simulink model "BlocksammlungJan2024_R2020"  (R2020a)
settings: Solver=ode45  StartTime=0.0  StopTime=10.0  RelTol=1e-3  EnableMultiTasking=on
undefined symbols (not defined in the file or in its folder): DiscIntNeverNeededParam, Kd, Ki, Kp, ta
libraries: simulink x13, dspxfrm3 x1
(part 1 of 2)
settings Model: Creator=METZLER  LastModifiedBy=PM
settings DataIOCC: LimitDataPoints=on  SaveFormat=Array  ReturnWorkspaceOutputs=off
settings OptimizationCC: LifeSpan=inf
settings DebuggingCC: SolverPrmCheckMsg=warning  PregeneratedLibrarySubsystemCodeDiagnostic=none  SFUnexpectedBacktrackingDiag=warning  SFNoUnconditionalDefaultTransitionDiag=warning  SFExecutionAtInitializationDiag=none  ArithmeticOperatorsInVariantConditions=warning
settings HardwareCC: ProdBitPerPointer=32  ProdBitPerSizeT=32  ProdBitPerPtrDiffT=32  ProdLargestAtomicFloat=None  ProdIntDivRoundTo=Undefined  ProdEndianess=Unspecified  ProdWordSize=32  ProdHWDeviceType=32-bit Generic
settings ModelReferenceCC: PropagateSignalLabelsOutOfModel=off
settings SFSimCC: SimUseLocalCustomCode=off  CustomCodeUndefinedFunction=UseInterfaceOnly
settings RTWCC: RTWUseLocalCustomCode=off
settings CodeAppCC: StateflowObjectComments=on
settings GRTTargetCC: TargetLangStandard=C89/C90 (ANSI)
settings ConfigComp: CovMetricSettings=dw  CovSaveCumulativeToWorkspaceVar=on  CovSaveSingleToWorkspaceVar=on  CovExternalEMLEnable=off  CovSFcnEnable=off

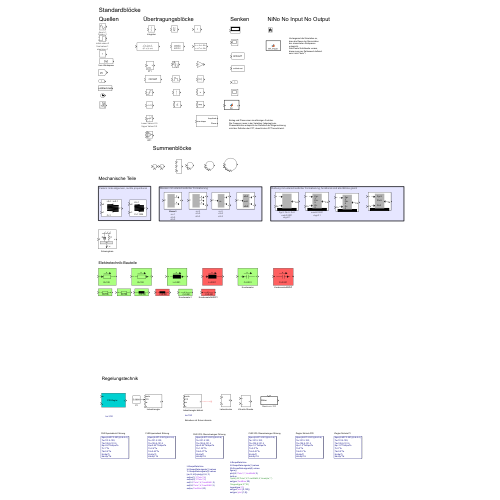
[thumbnail: Simulink's stored preview of the top-level diagram]
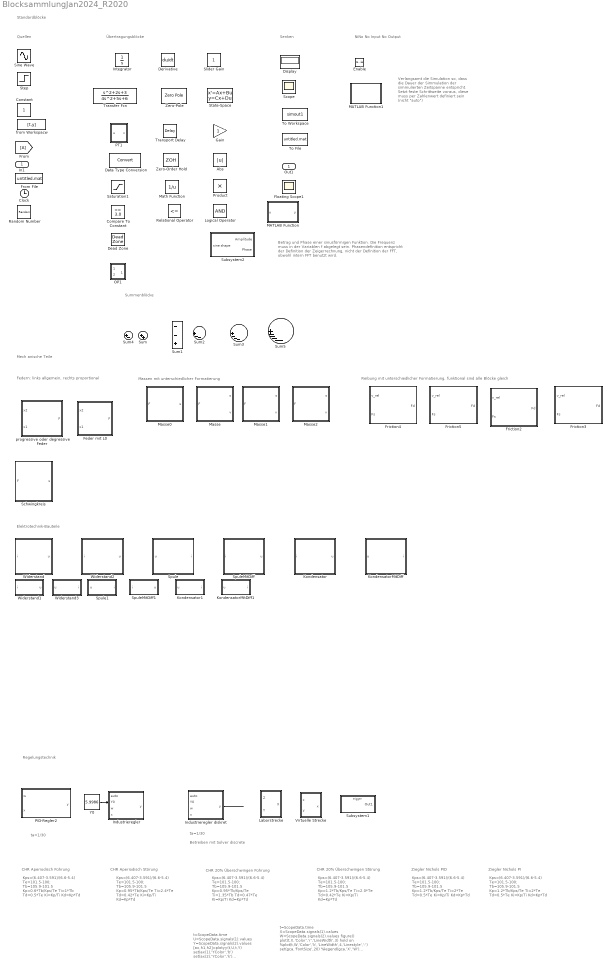
== system BlocksammlungJan2024_R2020 ==
  note: Elektrotechnik-Bauteile
  note: Federn: links allgemein, rechts proportional
  note: Reibung mit unterschiedlicher Formatierung, funktional sind alle Blöcke gleich
  note: Massen mit unterschiedlicher Formatierung
  note: Betrag und Phase einer sinusförmigen Funktion.
      | Die Frequenz muss in der Variablen f abgelegt sein.
      | Phasendefinition entspricht der Definition der Zeigerrechnung,
      | nicht der Definition der FFT, obwohl intern FFT benutzt wird.
  note: Verlangsamt die Simulation so, dass die Dauer der Simmulation der simmulierten Zeitspanne entspricht.
      | Setzt feste Schrittweite voraus, diese muss per Zahlenwert definiert sein (nicht "auto")
  note: t=ScopeData.time
      | X=ScopeData.signals(1).values
      | W=ScopeData.signals(2).values
      | figure()
      | plot(t,X,'Color','r','LineWidth',3)
      | hold on
      | %plot(t,W,'Color','k','LineWidth',4,'Linestyle',':')
      | set(gca,'FontSize',20)
      | %legend(gca,'X','W')
      | legend(gca,'X')
      | set(gca,'xlim',[0,150])
      | set(gca,'ylim',[1,8])
  note: Regelungstechnik
  note: Mech anische Teile
  note: Summenblöcke
  note: Senken
  note: Übertragungsblöcke
  note: Quellen
  note: Standardblöcke
  note: t=ScopeData.time
      | U=ScopeData.signals(1).values
      | Y=ScopeData.signals(2).values
      | [ax,h1,h2]=plotyy(t,U,t,Y)
      | set(ax(1),'YColor','b')
      | set(ax(2),'YColor','k')
      | set(h1,'Color','b','LineWidth',3)
      | set(h2,'Color','k','LineWidth',3)
      | set(ax,'FontSize',20)
  note: ta=1/30
  note: CHR Aperiodisch Führung
  note: CHR Aperiodisch Störung
  note: Kps=(6.407-3.591)/(6.6-5.4)
      | Te=101.5-100;
      | Tb=105.9-101.5
      | Kp=0.95*Tb/Kps/Te
      | Ti=1.35*Tb
      | Td=0.47*Te
      | Ki=Kp/Ti
      | Kd=Kp*Td
  note: Kps=(6.407-3.591)/(6.6-5.4)
      | Te=101.5-100;
      | Tb=105.9-101.5
      | Kp=0.6*Tb/Kps/Te
      | Ti=1*Tb
      | Td=0.5*Te
      | Ki=Kp/Ti
      | Kd=Kp*Td
  note: Kps=(6.407-3.591)/(6.6-5.4)
      | Te=101.5-100;
      | Tb=105.9-101.5
      | Kp=0.95*Tb/Kps/Te
      | Ti=2.4*Te
      | Td=0.42*Te
      | Ki=Kp/Ti
      | Kd=Kp*Td
  note: CHR 20% Überschwingen Führung
  note: Kps=(6.407-3.591)/(6.6-5.4)
      | Te=101.5-100;
      | Tb=105.9-101.5
      | Kp=1.2*Tb/Kps/Te
      | Ti=2.0*Te
      | Td=0.42*Te
      | Ki=Kp/Ti
      | Kd=Kp*Td
  note: CHR 20% Überschwingen Störung
  note: Ziegler Nichols PID
  note: Kps=(6.407-3.591)/(6.6-5.4)
      | Te=101.5-100;
      | Tb=105.9-101.5
      | Kp=1.2*Tb/Kps/Te
      | Ti=2*Te
      | Td=0.5*Te
      | Ki=Kp/Ti
      | Kd=Kp*Td
  note: NiNo No Input No Output
  note: Kps=(6.407-3.591)/(6.6-5.4)
      | Te=101.5-100;
      | Tb=105.9-101.5
      | Kp=1.2*Tb/Kps/Te
      | Ti=2*Te
      | Td=0.5*Te
      | Ki=Kp/Ti
      | Kd=Kp*Td
  note: Ziegler Nichols PI
  note: ta=1/30
  note: Betreiben mit Solver discrete
  In1 : Inport
  Enable : EnablePort
  " Feder mit L0" : Subsystem  mask{C=1.123456, L0=1}
      mask prompts: C "Spring Constant C [N/m]"; L0 "Length of Spring if no force is applied L0 [m]"
      mask help:
      | If no force F is applied, the spring has the length L0.
      |
      | F=C*sign(x2-x1-L0)*((x2-x1-L0)
      mask Display:
      | plot(20,0)
      | plot(90,100)
      | plot([60,60],[25,30])
      | plot([60,80],[30,32])
      | plot([80,40],[32,36])
      | plot([40,80],[36,40])
      | plot([80,40],[40,44])
      | plot([40,80],[44,48])
      | plot([80,40],[48,52])
      | plot([40,80],[52,56])
      | plot([80,40],[56,60])
      | plot([40,80],[60,64])
      | plot([80,40],[64,68])
      | plot([40,60],[68,70])
      | plot([60,60],[70,75])
      | 
      | 
      | port_label ('output',1,'F')
      | port_label ('input',1,'x2')
      | port_label ('input',2,'x1')
      | 
      | text(40,10,['C=',num2str(C)])
      | text(40,90,['L0=',num2str(L0)])
  " progressive oder degressive Feder" : Subsystem  mask{C=1, L0=1, Kappa=0.1}
      mask prompts: C "Federkonstante C [N/m]"; L0 "Entspannte Länge L0 [m]"; Kappa "Exponent Kappa"
      mask help:
      | Wenn keine Kraft wirkt, hat die Feder die Länge L0.
      | Progressive Feder: Kappa >0
      | Degressive Feder: Kappa <0
      | F=C*sign(x2-x1-L0)*abs(x2-x1-L0)^Kappa
      mask Display:
      | plot(20,0)
      | plot(90,100)
      | plot([60,60],[25,30])
      | plot([60,80],[30,32])
      | plot([80,40],[32,36])
      | plot([40,80],[36,40])
      | plot([80,40],[40,44])
      | plot([40,80],[44,48])
      | plot([80,40],[48,52])
      | plot([40,80],[52,56])
      | plot([80,40],[56,60])
      | plot([40,80],[60,64])
      | plot([80,40],[64,68])
      | plot([40,60],[68,70])
      | plot([60,60],[70,75])
      | 
      | 
      | port_label ('output',1,'F')
      | port_label ('input',1,'x2')
      | port_label ('input',2,'x1')
      | text(40,10,['C=',num2str(C)])
      | text(40,90,['L0=',num2str(L0),'  k=',num2str(Kappa)])
  Abs : Abs
  Clock : Clock
  Compare To Constant : simulink/Logic and Bit Operations/Compare To Constant  relop=<=  const=3.0  OutDataTypeStr=boolean
  Constant : Constant
  Data Type Conversion : DataTypeConversion
  Dead Zone : DeadZone  SaturateOnIntegerOverflow=on
      settings: AttributesFormatString=|
      | Lower Value=%<LowerValue>
      | Upper Value=%<UpperValue>
  Derivative : Derivative
  Display : Display
  Floating Scope1 : Scope
      settings: Floating=on
  Friction2 : Subsystem  mask{Fg=3, Fh=5, vhg=0.1, D=0, vsd=0.0001}
      mask prompts: Fg "Gleitreibung Fg"; Fh "Haftreibung Fh"; vhg "Übergangsbreite zwischen Haft- und Gleitreibung vhg"; D "Dämpfung D  (viskose Reibung)"; vsd "Übergangsbreite zwischen statischer und dynamischer Reibung"
      mask help:
      | Berechnet in Abhängigkeit von der Geschwindigkeit relativ zur Umgebung die Reibung eines Körpers.
      | Zunächst gibt es die statischer Reibung bei v=0 (Kraft entgegen der Summe der äußeren Kräfte ohne Fn) und die dynamische Reibung bei v<>0 (Kraft entgegen der Geschwindigkeit). Der Übergang zwischen beiden wird exponentiell verstetigt mit vsd als Übergangsbreite.
      | Dann gibt es im dynamischen noch mal einen Übergang zwischen Haftreibung (v klein) und Gleitreibung (v größer) mit vhg als Übergangsbreite. Für höhere Geschwindigkeiten macht sich noch die viskose Reibung D*v bemerkbar.
      mask Display:
      | plot(0,0)
      | plot(100,100)
      | 
      | 
      | patch([10 10 90 90],[0 10 10 0],[0 0 0 ])
      | patch([30 30 70 70],[11 90 90 11],[0.7 0.7 0.7 ])
      | plot([15 28],[75 75])
      | patch([25 25 30],[69 79 74],[0 0 0])
      | plot([71 85],[48 48])
      | patch([70 75 75],[48 43 53],[0 0 0])
      | plot([15 28],[25 25])
      | patch([25 25 30],[20 30 25],[0 0 0])
      | port_label ('output',1,'Fd')
      | port_label ('input',1,'v')
      | port_label ('input',2,'Fs')
      | text(40,80,'Fg=')
      | text(40,70,num2str(Fg))
      | %text(40,80,['Fg=',num2str(Fg)])
      | %text(40,55,['Fh=',num2str(Fh)])
      | text(40,55,'Fh=')
      | text(40,45,num2str(Fh))
      | text(40,30,'D=')
      | text(40,20,num2str(D))
  Friction3 : Subsystem  mask{Fg=3, Fh=5, vhg=0.1, D=0, vsd=0.0001}
      mask prompts: Fg "Gleitreibung Fg"; Fh "Haftreibung Fh"; vhg "Übergangsbreite zwischen Haft- und Gleitreibung vhg"; D "Dämpfung D  (viskose Reibung)"; vsd "Übergangsbreite zwischen statischer und dynamischer Reibung"
      mask help:
      | Berechnet in Abhängigkeit von der Geschwindigkeit relativ zur Umgebung die Reibung eines Körpers.
      | Zunächst gibt es die statischer Reibung bei v=0 (Kraft entgegen der Summe der äußeren Kräfte ohne Fn) und die dynamische Reibung bei v<>0 (Kraft entgegen der Geschwindigkeit). Der Übergang zwischen beiden wird exponentiell verstetigt mit vsd als Übergangsbreite.
      | Dann gibt es im dynamischen noch mal einen Übergang zwischen Haftreibung (v klein) und Gleitreibung (v größer) mit vhg als Übergangsbreite. Für höhere Geschwindigkeiten macht sich noch die viskose Reibung D*v bemerkbar.
      mask Display:
      | plot(0,0)
      | plot(100,100)
      | 
      | 
      | patch([10 10 90 90],[0 10 10 0],[0 0 0 ])
      | patch([30 30 70 70],[11 90 90 11],[0.7 0.7 0.7 ])
      | plot([15 28],[75 75])
      | patch([25 25 30],[69 79 74],[0 0 0])
      | plot([71 85],[48 48])
      | patch([70 75 75],[48 43 53],[0 0 0])
      | plot([15 28],[25 25])
      | patch([25 25 30],[20 30 25],[0 0 0])
      | port_label ('output',1,'Fd')
      | port_label ('input',1,'v')
      | port_label ('input',2,'Fs')
      | text(40,80,['Fg=',num2str(Fg)])
      | text(40,55,['Fh=',num2str(Fh)])
      | text(40,30,['D=',num2str(D)])
      | %text(40,80,'Fg=')
      | %text(40,70,num2str(Fg))
      | %text(40,55,'Fh=')
      | %text(40,45,num2str(Fh))
      | %text(40,30,'D=')
      | %text(40,20,num2str(D))
  Friction4 : Subsystem  mask{Fg=3, Fh=5, vhg=0.1, D=0, vsd=0.0001}
      mask prompts: Fg "Gleitreibung Fg"; Fh "Haftreibung Fh"; vhg "Übergangsbreite zwischen Haft- und Gleitreibung vhg"; D "Dämpfung D  (viskose Reibung)"; vsd "Übergangsbreite zwischen statischer und dynamischer Reibung"
      mask help:
      | Berechnet in Abhängigkeit von der Geschwindigkeit relativ zur Umgebung die Reibung eines Körpers.
      | Zunächst gibt es die statischer Reibung bei v=0 (Kraft entgegen der Summe der äußeren Kräfte ohne Fn) und die dynamische Reibung bei v<>0 (Kraft entgegen der Geschwindigkeit). Der Übergang zwischen beiden wird exponentiell verstetigt mit vsd als Übergangsbreite.
      | Dann gibt es im dynamischen noch mal einen Übergang zwischen Haftreibung (v klein) und Gleitreibung (v größer) mit vhg als Übergangsbreite. Für höhere Geschwindigkeiten macht sich noch die viskose Reibung D*v bemerkbar.
      settings: AttributesFormatString=|
      | Fg=%<Fg>  Fh=%<Fh>  D=%<D>\nvsd=%<vsd>
      | vhg=%<vhg>
      mask Display:
      | plot(0,0)
      | plot(100,100)
      | 
      | 
      | patch([10 10 90 90],[0 10 10 0],[0 0 0 ])
      | patch([30 30 70 70],[11 90 90 11],[0.7 0.7 0.7 ])
      | plot([15 28],[75 75])
      | patch([25 25 30],[69 79 74],[0 0 0])
      | plot([71 85],[48 48])
      | patch([70 75 75],[48 43 53],[0 0 0])
      | plot([15 28],[25 25])
      | patch([25 25 30],[20 30 25],[0 0 0])
      | port_label ('output',1,'Fd')
      | port_label ('input',1,'v')
      | port_label ('input',2,'Fs')
  Friction5 : Subsystem  mask{Fg=3, Fh=5, vhg=0.1, D=0, vsd=0.0001}
      mask prompts: Fg "Gleitreibung Fg"; Fh "Haftreibung Fh"; vhg "Übergangsbreite zwischen Haft- und Gleitreibung vhg"; D "Dämpfung D  (viskose Reibung)"; vsd "Übergangsbreite zwischen statischer und dynamischer Reibung"
      mask help:
      | Berechnet in Abhängigkeit von der Geschwindigkeit relativ zur Umgebung die Reibung eines Körpers.
      | Zunächst gibt es die statischer Reibung bei v=0 (Kraft entgegen der Summe der äußeren Kräfte ohne Fn) und die dynamische Reibung bei v<>0 (Kraft entgegen der Geschwindigkeit). Der Übergang zwischen beiden wird exponentiell verstetigt mit vsd als Übergangsbreite.
      | Dann gibt es im dynamischen noch mal einen Übergang zwischen Haftreibung (v klein) und Gleitreibung (v größer) mit vhg als Übergangsbreite. Für höhere Geschwindigkeiten macht sich noch die viskose Reibung D*v bemerkbar.
      settings: AttributesFormatString=|
      | nvsd=%<vsd>
      | vhg=%<vhg>
      mask Display:
      | plot(0,0)
      | plot(100,100)
      | 
      | 
      | patch([10 10 90 90],[0 10 10 0],[0 0 0 ])
      | patch([30 30 70 70],[11 90 90 11],[0.7 0.7 0.7 ])
      | plot([15 28],[75 75])
      | patch([25 25 30],[69 79 74],[0 0 0])
      | plot([71 85],[48 48])
      | patch([70 75 75],[48 43 53],[0 0 0])
      | plot([15 28],[25 25])
      | patch([25 25 30],[20 30 25],[0 0 0])
      | port_label ('output',1,'Fd')
      | port_label ('input',1,'v')
      | port_label ('input',2,'Fs')
      | text(40,80,'Fg=')
      | text(40,70,num2str(Fg))
      | %text(40,80,['Fg=',num2str(Fg)])
      | %text(40,55,['Fh=',num2str(Fh)])
      | text(40,55,'Fh=')
      | text(40,45,num2str(Fh))
      | text(40,30,'D=')
      | text(40,20,num2str(D))
  From File : FromFile  SampleTime=0
  Gain : Gain
  Industrieregler : Subsystem  mask{Kp=Kp, Ki=Ki, Kd=Kd, T=0.1, Ts=0.1, E0_auf_I=on, E0_auf_P=on, Stossfrei=on}
      mask prompts: T "Zeitkonstante   DT1-Glied"; Ts "Dauer Ts der stossfreien Umschaltung (>0)"; E0_auf_I "Integrier-Pfad sieht Anfangsfehler"; E0_auf_P "Proportional-Pfad sieht Anfangsfehler"; Stossfrei "Stossfreie Umschaltung"
      mask help:
      | Industrieregler. Zum Korrekten Hin- und Herschalten zwischen Hand und Automatik muss Y0 aus einer Konstantquelle namens Y0 kommen,
      | Diese Variante funktioniert auch mit variabler Schrittweite.
      | Wegen den kontinuierlichen Zuständen funktioniert diese Variante aber nicht mit Hardwaretargets.
      mask Display:
      | port_label('input',1,'auto');
      | port_label('input',2,'Y0');
      | port_label('input',3,'w');
      | port_label('input',4,'x');
      | port_label('output',1,'y');
  Industrieregler diskret : Subsystem  mask{Kp=0.885, Ki=0.17, Kd=0.99, T=1, Ts=1, E0_auf_I=on, E0_auf_P=off, Stossfrei=on}
      mask prompts: T "Zeitkonstante   DT1-Glied"; Ts "Dauer Ts der stossfreien Umschaltung (>0)"; E0_auf_I "Integrier-Pfad sieht Anfangsfehler"; E0_auf_P "Proportional-Pfad sieht Anfangsfehler"; Stossfrei "Stossfreie Umschaltung"
      mask help:
      | Industrieregler.
      | Zum Korrekten Hin- und Herschalten zwischen Hand und Automatik muss Y0 aus einer Konstantquelle namens Y0 kommen,
      | Diese Variante funktioniertnur mit fester Schrittweite.
      | Diese Variante funktioniert auch mit Hardwaretargets.
      mask Display:
      | port_label('input',1,'auto');
      | port_label('input',2,'Y0');
      | port_label('input',3,'w');
      | port_label('input',4,'x');
      | port_label('output',1,'y');
  Integrator : Integrator
  Kondensator : Subsystem  mask{C=1E-3}
      mask prompts: C "Kappazität C [F]"
      mask help:
      | Kapazität
      | Eingang ist u, Ausgang ist i.
      | i=1/C * integral(u)
      mask Display:
      | plot(0,0)
      | plot(100,100)
      | plot([0 0],[1 1]) %Umschalten auf dicke Linien
      | %patch([30 30 70 70 30],[40 60 60 40 40],[0,0,0])
      | plot([45 45],[40 60])
      | plot([55 55],[40 60])
      | plot([15 45],[50 50])
      | patch([25,32,25],[45,50,55],[0,0,0])
      | plot([55 85],[50 50])
      | plot([30 70],[70 70])
      | patch([63 70 63],[65 70 75], [0,0,0])
      | text(45,80,['u'])
      | 
      | text(30,20,['C=',num2str(C)])
      | 
      | 
      | 
      | port_label ('output',1,'u')
      | port_label ('input',1,'i')
  Kondensator1 : Subsystem  mask{C=1E-3}
      mask prompts: C "Kappazität C [F]"
      mask help:
      | Kapazität
      | Eingang ist u, Ausgang ist i.
      | i=1/C * integral(u)
      mask Display:
      | plot(0,0)
      | plot(100,100)
      | plot([0 0],[1 1]) %Umschalten auf dicke Linien
      | %patch([30 30 70 70 30],[40 60 60 40 40],[0,0,0])
      | plot([45 45],[40 60])
      | plot([55 55],[40 60])
      | plot([15 45],[50 50])
      | 
      | plot([55 85],[50 50])
      | 
      | 
      | 
      | text(30,19,['C=',num2str(C)])
      | 
      | 
      | 
      | port_label ('output',1,'u')
      | port_label ('input',1,'i')
  KondensatorMitDiff : Subsystem  mask{C=1E-3}
      mask prompts: C "Kappazität C [F]"
      mask help:
      | Kapazität
      | Eingang ist u, Ausgang ist i.
      | i=C*u'
      | Wegen Diff-Block nicht für jeden Solver geeignet.
      mask Display:
      | plot(0,0)
      | plot(100,100)
      | plot([0 0],[1 1]) %Umschalten auf dicke Linien
      | %patch([30 30 70 70 30],[40 60 60 40 40],[0,0,0])
      | plot([45 45],[40 60])
      | plot([55 55],[40 60])
      | plot([15 45],[50 50])
      | patch([70,77,70],[45,50,55],[0,0,0])
      | plot([55 85],[50 50])
      | plot([30 70],[70 70])
      | patch([63 70 63],[65 70 75], [0,0,0])
      | text(45,80,['u'])
      | 
      | text(30,20,['C=',num2str(C)])
      | 
      | 
      | 
      | port_label ('output',1,'i')
      | port_label ('input',1,'u')
  KondensatorMitDiff1 : Subsystem  mask{C=1E-3}
      mask prompts: C "Kappazität C [F]"
      mask help:
      | Kapazität
      | Eingang ist u, Ausgang ist i.
      | i=C*u'
      | Wegen Diff-Block nicht für jeden Solver geeignet.
      mask Display:
      | plot(0,0)
      | plot(100,100)
      | plot([0 0],[1 1]) %Umschalten auf dicke Linien
      | %patch([30 30 70 70 30],[40 60 60 40 40],[0,0,0])
      | plot([45 45],[40 60])
      | plot([55 55],[40 60])
      | plot([15 45],[50 50])
      | 
      | plot([55 85],[50 50])
      | 
      | 
      | 
      | text(30,19,['C=',num2str(C)])
      | 
      | 
      | 
      | port_label ('output',1,'i')
      | port_label ('input',1,'u')
  Laborstrecke : Subsystem
  Logical Operator : Logic  AllPortsSameDT=off  OutDataTypeStr=boolean
  MATLAB Function : MATLAB Function  TreatAsAtomicUnit=on
  MATLAB Function1 : MATLAB Function  TreatAsAtomicUnit=on
  Masse : Subsystem  mask{m=2, v0=0, s0=3}
      mask prompts: m "Masse m"; v0 "Anfangsgeschwindigkeit v_0"; s0 "Anfangsposition s_0"
      mask help:
      | Calculates the position s and the velocity v of a mass as a function of the Force F and the initial velocity v_0 and initial position s_0.
      | Berechnet die Position und die Geschwindigkeit eines Köpers mit der Masse m. Auf den Köper wirkt die Kraft F. Die Anfangsposition ist s_0, die Anfangsgeschwindigkeit ist v_0.
      settings: AttributesFormatString=m=%<m>\nv0=%<v0>\ns0=%<s0>
      mask Display:
      | plot(0,0)
      | plot(100,100)
      | patch([20 20 60 60],[10 90 90 10],[0.7,0.7,0.7])
      | plot([60 80],[70 70])
      | patch([80 80 85],[65 75 70],[0 0 0])
      | text(70,80,'s')
      | plot([60 80],[50 50])
      | patch([80 80 85],[45 55 50],[0 0 0])
      | text(70,60,'F')
      | plot([60 80],[30 30])
      | patch([80 80 85],[25 35 30],[0 0 0])
      | text(70,40,'v')
      | port_label ('output',1,'s')
      | port_label ('output',2,'v')
      | port_label ('input',1,'F')
  Masse0 : Subsystem  mask(Starrer Körper){m=1, v0=0, s0=0}
      mask prompts: m "Masse m"; v0 "Anfangsgeschwindigkeit v0"; s0 "Anfangsposition s0"
      mask help: Berechnet die Position eines Körpers als Funktion der auf ihn wirkenden Kraft F, seiner Masse m, der Anfangsgeschwindigkeit v0 und der Anfangsposition s0.
      settings: AttributesFormatString=m=%<m>\nv0=%<v0>\ns0=%<s0>
      mask Help:
      | Die Position x eines starren Körpers der Masse m berechnet sich aus:
      | F=m*X''
      | 
      | Erstellt von Patrick Metzler für Hochschule RheinMain.
      mask Display:
      | plot(0,0)
      | plot(100,100)
      | patch([20 20 60 60],[10 90 90 10],[0.7,0.7,0.7])
      | plot([60 80],[70 70])
      | patch([80 80 85],[65 75 70],[0 0 0])
      | text(70,80,'F')
      | plot([60 80],[30 30])
      | patch([80 80 85],[25 35 30],[0 0 0])
      | text(70,40,'s')
      | port_label ('output',1,'s')
      | port_label ('input',1,'F')
  Masse1 : Subsystem  mask{m=2, v0=0, s0=3}
      mask prompts: m "Masse m"; v0 "Anfangsgeschwindigkeit v_0"; s0 "Anfangsposition s_0"
      mask help:
      | Calculates the position s and the velocity v of a mass as a function of the Force F and the initial velocity v_0 and initial position s_0.
      | Berechnet die Position und die Geschwindigkeit eines Köpers mit der Masse m. Auf den Köper wirkt die Kraft F. Die Anfangsposition ist s_0, die Anfangsgeschwindigkeit ist v_0.
      settings: AttributesFormatString=m=%<m>\nv0=%<v0>\ns0=%<s0>
      mask Display:
      | plot(0,0)
      | plot(100,100)
      | patch([35 35 70 70],[10 90 90 10],[0.7,0.7,0.7])
      | text(45,50,'m')
      | plot([70 80],[70 70])
      | patch([80 80 85],[65 75 70],[0 0 0])
      | plot([15 35],[50 50])
      | patch([30 30 35],[45 55 50],[0 0 0])
      | plot([70 80],[30 30])
      | patch([80 80 85],[25 35 30],[0 0 0])
      | port_label ('output',1,'s')
      | port_label ('output',2,'v')
      | port_label ('input',1,'F')
  Masse2 : Subsystem  mask{m=2, v0=0, s0=3}
      mask prompts: m "Masse m"; v0 "Anfangsgeschwindigkeit v_0"; s0 "Anfangsposition s_0"
      mask help:
      | Calculates the position s and the velocity v of a mass as a function of the Force F and the initial velocity v_0 and initial position s_0.
      | Berechnet die Position und die Geschwindigkeit eines Köpers mit der Masse m. Auf den Köper wirkt die Kraft F. Die Anfangsposition ist s_0, die Anfangsgeschwindigkeit ist v_0.
      mask Display:
      | plot(0,0)
      | plot(100,100)
      | patch([35 35 70 70],[10 90 90 10],[0.7,0.7,0.7])
      | text(40,80,['s0=',num2str(s0)])
      | text(40,50,['m=',num2str(m)])
      | text(40,20,['v0=',num2str(v0)])
      | plot([70 80],[70 70])
      | patch([80 80 85],[65 75 70],[0 0 0])
      | plot([15 35],[50 50])
      | patch([30 30 35],[45 55 50],[0 0 0])
      | plot([70 80],[30 30])
      | patch([80 80 85],[25 35 30],[0 0 0])
      | port_label ('output',1,'s')
      | port_label ('output',2,'v')
      | port_label ('input',1,'F')
  Math Function : Math  Operator=reciprocal  SignedPower=on  SaturateOnIntegerOverflow=on
  OP1 : Subsystem  mask{k0=1E5, fg=100000}
      mask prompts: k0 "Open Loop Gain [V/V]"; fg "Open Loop Band Width [Hz]"
      mask init:
      | set_param(gcb,'MaskHideContents','off')
      mask Display:
      | color('black')
      | patch([0.2 0.2 0.8 0.2],[0.05 0.95 0.5 0.051],[0.9 0.9 0.9 ])
      | plot([0.2 0.2],[0.05 0.95])% Senkrecht Gehäuse
      | 
      | plot([0.2 0.8],[0.95 0.5])% Gehäuse oben schräg
      | plot([0.2 0.8],[0.051 0.5])% Gehäuse unten schräg
      | plot([0.0 0.2],[0.75 0.75])% Leiterbahn Plus
      | plot([0.0 0.2],[0.25 0.25])% Leiterbahn Minus
      | plot([0.8 1],[0.5 0.5])% Leiterbahn ua
      | text(0.29,0.76,'+')
      | text(0.29,0.28,'-')
      | %patch([0.1 0.9 0.9 0.1 0.1],[0.1 0.1 0.9 0.9 0.1],[0 0 0 ])
  PID-Regler2 : Subsystem  mask{Kp=1, Ki=1, Kd=1, T=0.1}
      mask prompts: T "T  Zeitkonstante des PT1-Glieds vor dem D-Glied"
      mask help: Ein einfacher PID-Regler
      mask Display:
      | IconText='';
      | if ~strcmp(get_param(gcb,'Kp'),'0')
      |     IconText=strcat(IconText,'P');
      | end
      | if ~strcmp(get_param(gcb,'Ki'),'0')
      |    IconText=strcat(IconText,'I');
      | end
      | if ~strcmp(get_param(gcb,'Kd'),'0')
      |     IconText=strcat(IconText,'D');
      | end
      | IconText=strcat(IconText,'-Regler')
      | plot(0,0)
      | plot(100,100)
      | text(25,50,IconText)
      | port_label ('output',1,'y')
      | port_label ('input',1,'w')
      | port_label ('input',2,'x')
  PT1 : Subsystem  mask{k=1, T=1}
      mask prompts: k "Verstärkung"; T "Zeitkonstante"
      mask help: PT1-Glied
      mask Display:
      | plot(0,0)
      | plot(100,100)
      | text(20,20,'PT1')
      | port_label ('output',1,'v')
      | port_label ('input',1,'u')
  Product : Product
  Random Number : RandomNumber  SampleTime=0.1
  Relational Operator : RelationalOperator  Operator=<=  OutDataTypeStr=boolean  RndMeth=Simplest
  Saturation1 : Saturate
  Schwingkreis : Subsystem  mask{v0=0, C=1, D=1, m=1}
      mask prompts: v0 "Anfangsgeschwindigkeit [m/s]"; C "Federkonstante [N/m]"; D "Dämpfung [Ns/m]"; m "Masse [kg]"
      mask help:
      | Ein einfacher Schwingkreis erregt durch die Kraft F antwortet mit der Position x.
      | Die Kraft wird in Newton erwartet, die Position wird in Metern ausgegeben.
      mask Display:
      | plot(0,0)
      | plot(100,100)
      | %innerhalb einer Make hat das plot-commando
      | %keine modifier.
      | %Durch zweimal gleiche Koordinaten am Anfang des
      | %plot-Kommandos wird auf dicke Linie umgeschaltet.
      | 
      | plot([20,20 70],[80,80 80])
      | plot([30 40],[80 90])
      | plot([45 55],[80 90])
      | plot([60 70],[80 90])
      | 
      | patch([30 42 42 30],[55 55 58 58],[0 0 0 ])
      | plot([28 28],[63 50])
      | plot([42 42],[63 50])
      | plot([28 42],[50 50])
      | plot([35 35],[60 80])
      | plot([35 35],[50 30])
      | 
      | patch([14 78 78 14],[26 26 38 38],[0.9 0.9 0.9])
      | text(44,33,'m')
      | plot([10 80],[25 25])
      | plot([10 80],[39 39])
      | plot([10 10],[25 39])
      | plot([80 80],[25 39])
      | 
      | plot([60 60],[80 70])
      | plot([60 55],[70 68])
      | plot([55 65],[68 64])
      | plot([65 55],[64 60])
      | plot([55 65],[60 55])
      | plot([55 65],[51 55])
      | plot([55 60],[51 49])
      | plot([60 60],[49 39])
      | 
      | plot([45 45],[25 5])
      | 
      | patch([43 46 49],[10 5 10],[0  0 0])
      | 
      | text(50,15,'F, x')
      | text(70,60,'C')
      | text(20,60,'D')
      | 
      | port_label ('output',1,'x')
      | port_label ('input',1,'F')
  Scope : Scope
  Sine Wave : Sin  SampleTime=0
      settings: AttributesFormatString=|
      | Ampl.=%<Amplitude>
      | Frequ.=%<Frequency>
      | Offset=%<Offset>
      | Phase=%<Phase>
  Slider Gain : simulink/Math Operations/Slider Gain  gain=1  low=0  high=2
  Spule : Subsystem  mask{L=1E-3}
      mask prompts: L "Induktivität L [H]"
      mask help:
      | Induktivität:
      | Eingang ist u, Ausgang ist i.
      mask Display:
      | plot(0,0)
      | plot(100,100)
      | plot([0 0],[1 1]) %Umschalten auf dicke Linien
      | patch([30 30 70 70 30],[40 60 60 40 40],[0,0,0])
      | plot([15 30],[50 50])
      | patch([75,82,75],[45,50,55],[0,0,0])
      | plot([70 88],[50 50])
      | plot([30 70],[70 70])
      | patch([63 70 63],[65 70 75], [0,0,0])
      | text(45,80,['u'])
      | 
      | text(30,20,['L=',num2str(L)])
      | 
      | 
      | 
      | port_label ('output',1,'i')
      | port_label ('input',1,'u')
  Spule1 : Subsystem  mask{L=1E-3}
      mask prompts: L "Induktivität L [H]"
      mask help:
      | Induktivität:
      | Eingang ist u, Ausgang ist i.
      mask Display:
      | plot(0,0)
      | plot(100,100)
      | plot([0 0],[1 1]) %Umschalten auf dicke Linien
      | patch([30 30 70 70 30],[35 65 65 35 35],[0,0,0])
      | plot([15 30],[50 50])
      | plot([70 88],[50 50])
      | text(30,20,['L=',num2str(L)])
      | port_label ('output',1,'i')
      | port_label ('input',1,'u')
  SpuleMitDiff : Subsystem  mask{L=1E-3}
      mask prompts: L "Induktivität L [H]"
      mask help:
      | Induktivität
      | Eingang ist i, Ausgang ist u.
      | u=L*i'
      | Wegen Diff-Block nicht für alle Solver geeignet.
      mask Display:
      | plot(0,0)
      | plot(100,100)
      | plot([0 0],[1 1]) %Umschalten auf dicke Linien
      | patch([30 30 70 70 30],[40 60 60 40 40],[0,0,0])
      | plot([15 30],[50 50])
      | patch([20,27,20],[45,50,55],[0,0,0])
      | plot([70 88],[50 50])
      | plot([30 70],[70 70])
      | patch([63 70 63],[65 70 75], [0,0,0])
      | text(45,80,['u'])
      | 
      | text(30,20,['L=',num2str(L)])
      | 
      | 
      | 
      | port_label ('output',1,'u')
      | port_label ('input',1,'i')
  SpuleMitDiff1 : Subsystem  mask{L=1E-3}
      mask prompts: L "Induktivität L [H]"
      mask help:
      | Induktivität
      | Eingang ist i, Ausgang ist u.
      | u=L*i'
      | Wegen Diff-Block nicht für alle Solver geeignet.
      mask Display:
      | plot(0,0)
      | plot(100,100)
      | plot([0 0],[1 1]) %Umschalten auf dicke Linien
      | patch([30 30 70 70 30],[35 65 65 35 35],[0,0,0])
      | plot([15 30],[50 50])
      | 
      | plot([70 85],[50 50])
      | 
      | 
      | text(30,20,['L=',num2str(L)])
      | 
      | 
      | 
      | port_label ('output',1,'u')
      | port_label ('input',1,'i')
  State-Space : StateSpace  InitialCondition=0
  Step : Step  SampleTime=0
      settings: AttributesFormatString=initial value=%<Before>\nfinal value=%<After>\nstep time=%<Time>
  Subsystem1 : Subsystem  mask(Counter){Maximum=100}
      mask prompts: Maximum "Maximum Count, when this is reached, reset to zero"
      mask help:
      | Counts with each rising trigger till maximum is reached.
      | Then starts all over with 0.
      settings: AttributesFormatString=Maximum=%<Maximum>
      mask Display: text(1,20,'Zähler')
  Subsystem2 : Subsystem
  Sum : Sum  Inputs=|++
  Sum1 : Sum  Inputs=--+
  Sum2 : Sum  Inputs=||+--
  Sum3 : Sum  Inputs=|||+---
  Sum4 : Sum  Inputs=|+-
  Sum5 : Sum  Inputs=|||||+-----
  To File : ToFile  SaveFormat=Timeseries
  To Workspace : ToWorkspace  VariableName=simout1  SaveFormat=Structure  SampleTime=-1
  Transfer Fcn : TransferFcn  Numerator=[1 2 3]  Denominator=[4 5 6]
  Transport Delay : TransportDelay
  Virtuelle Strecke : Subsystem
  Widerstand : Subsystem  mask{R=100}
      mask prompts: R "Widerstand [Ohm]"
      mask help: Ohm'scher Widerstand, Eingang ist i, Ausgang ist u.
      mask Display:
      | plot(0,0)
      | plot(100,100)
      | plot([0 0],[1 1]) %Umschalten auf dicke Linien
      | plot([30 30 70 70 30],[40 60 60 40 40])
      | plot([10 30],[50 50])
      | patch([18,25,18],[45,50,55],[0,0,0])
      | plot([70 89],[50 50])
      | plot([30 70],[70 70])
      | patch([63 70 63],[65 70 75], [0,0,0])
      | text(45,80,['u'])
      | 
      | text(30,20,['R=',num2str(R)])
      | 
      | 
      | 
      | port_label ('output',1,'u')
      | port_label ('input',1,'i')
  Widerstand1 : Subsystem  mask{R=100}
      mask prompts: R "Widerstand [Ohm]"
      mask help: Ohm'scher Widerstand, Eingang ist i, Ausgang ist u.
      mask Display:
      | plot(0,0)
      | plot(100,100)
      | plot([0 0],[1 1]) %Umschalten auf dicke Linien
      | plot([30 30 70 70 30],[35 65 65 35 35])
      | plot([15 30],[50 50])
      | plot([70 88],[50 50])
      | 
      | 
      | text(30,20,['R=',num2str(R)])
      | 
      | 
      | 
      | port_label ('output',1,'u')
      | port_label ('input',1,'i')
  Widerstand2 : Subsystem  mask{R=100}
      mask prompts: R "Widerstand [Ohm]"
      mask help: Ohm'scher Widerstand, Eingang ist u, Ausgang ist i.
      mask Display:
      | plot(0,0)
      | plot(100,100)
      | plot([0 0],[1 1]) %Umschalten auf dicke Linien
      | plot([30 30 70 70 30],[40 60 60 40 40])
      | plot([15 30],[50 50])
      | patch([75,82,75],[45,50,55],[0,0,0])
      | plot([70 88],[50 50])
      | plot([30 70],[70 70])
      | patch([63 70 63],[65 70 75], [0,0,0])
      | text(45,80,['u'])
      | 
      | text(30,20,['R=',num2str(R)])
      | 
      | 
      | 
      | port_label ('output',1,'i')
      | port_label ('input',1,'u')
  Widerstand3 : Subsystem  mask{R=100}
      mask prompts: R "Widerstand [Ohm]"
      mask help: Ohm'scher Widerstand, Eingang ist u, Ausgang ist i.
      mask Display:
      | plot(0,0)
      | plot(100,100)
      | plot([0 0],[1 1]) %Umschalten auf dicke Linien
      | plot([30 30 70 70 30],[35 65 65 35 35])
      | plot([15 30],[50 50])
      | plot([70 88],[50 50])
      | 
      | 
      | text(30,20,['R=',num2str(R)])
      | 
      | 
      | 
      | port_label ('output',1,'i')
      | port_label ('input',1,'u')
  Y0 : Constant  Value=5.9986
  Zero-Order Hold : ZeroOrderHold
  Zero-Pole : ZeroPole  Poles=[0 -1]
  from Workspacw : FromWorkspace  VariableName=[t,y]
  Out1 : Outport  VectorParamsAs1DForOutWhenUnconnected=off
  wires:
  Y0/1 -> Industrieregler/2(Y0)
  Industrieregler diskret/1(y) -> ?

== system BlocksammlungJan2024_R2020/ Feder mit L0 ==
  note: jutst use the sign function
  x2 : Inport
  x1 : Inport  Port=2
  Gain : Gain  Gain=C
  Lo : Constant  Value=L0
  Sum : Sum  Inputs=+--
  F : Outport  VectorParamsAs1DForOutWhenUnconnected=off
  wires:
  Gain/1 -> F/1
  Sum/1 -> Gain/1
  Lo/1 -> Sum/3
  x1/1 -> Sum/2
  x2/1 -> Sum/1

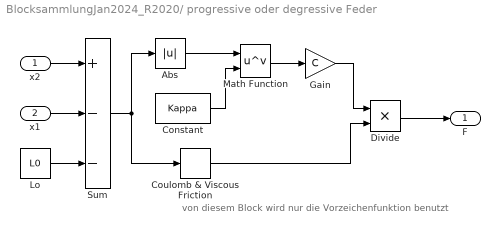
== system BlocksammlungJan2024_R2020/ progressive oder degressive Feder ==
  note: von diesem Block wird nur die Vorzeichenfunktion benutzt
  x2 : Inport
  x1 : Inport  Port=2
  Abs : Abs
  Constant : Constant  Value=Kappa
  Coulomb & Viscous Friction : simulink/Discontinuities/Coulomb & Viscous Friction  offset=[1]  gain=0
  Divide : Product  Inputs=**
  Gain : Gain  Gain=C
  Lo : Constant  Value=L0
  Math Function : Math  Operator=pow  SignedPower=on  SaturateOnIntegerOverflow=on
  Sum : Sum  Inputs=+--
  F : Outport  VectorParamsAs1DForOutWhenUnconnected=off
  wires:
  Abs/1 -> Math Function/1
  Divide/1 -> F/1
  Coulomb & Viscous Friction/1 -> Divide/2
  Gain/1 -> Divide/1
  Math Function/1 -> Gain/1
  Lo/1 -> Sum/3
  x1/1 -> Sum/2
  x2/1 -> Sum/1
  Sum/1 -> Abs/1, Coulomb & Viscous Friction/1
  Constant/1 -> Math Function/2

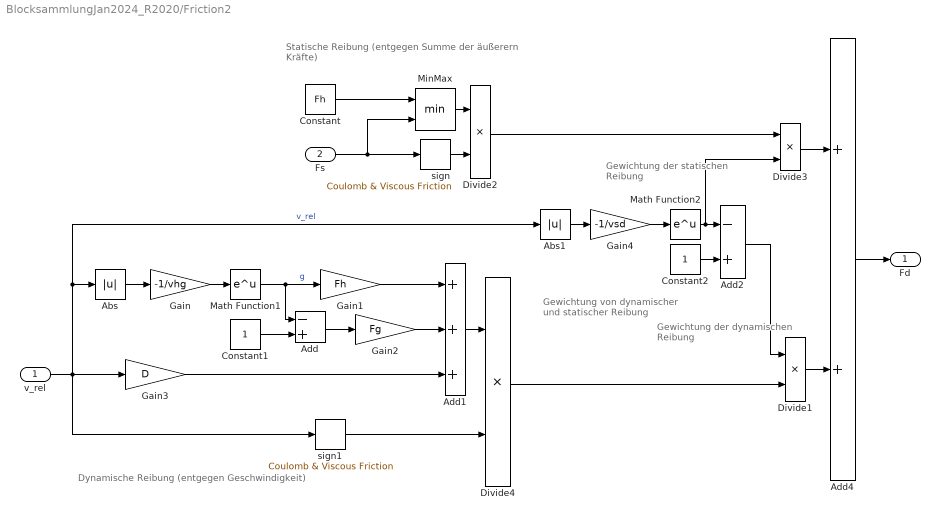
== system BlocksammlungJan2024_R2020/Friction2 ==
  note: Gewichtung von dynamischer
      |  und statischer Reibung
  note: Statische Reibung
      | (entgegen Summe der äußerern Kräfte)
  note: Dynamische Reibung (entgegen Geschwindigkeit)
  note: Gewichtung der
      | dynamischen Reibung
  note: Gewichtung der
      | statischen Reibung
  v_rel : Inport
  Fs : Inport  Port=2
  Abs : Abs
  Abs1 : Abs
  Add : Sum  Inputs=-+
  Add1 : Sum  Inputs=+++
  Add2 : Sum  Inputs=-+
  Add4 : Sum
  Constant : Constant  Value=Fh
  Constant1 : Constant
  Constant2 : Constant
  Divide{1..4} (4 alike) : Product  Inputs=**
  Gain : Gain  Gain=-1/vhg
  Gain1 : Gain  Gain=Fh
  Gain2 : Gain  Gain=Fg
  Gain3 : Gain  Gain=D
  Gain4 : Gain  Gain=-1/vsd
  Math Function1 : Math  SignedPower=on  SaturateOnIntegerOverflow=on
  Math Function2 : Math  SignedPower=on  SaturateOnIntegerOverflow=on
  MinMax : MinMax  Inputs=2
  sign : simulink/Discontinuities/Coulomb & Viscous Friction  offset=[1]  gain=0
  sign1 : simulink/Discontinuities/Coulomb & Viscous Friction  offset=[1]  gain=0
  Fd : Outport  VectorParamsAs1DForOutWhenUnconnected=off
  wires:
  Abs/1 -> Gain/1
  Gain/1 -> Math Function1/1
  Math Function1/1 -> Add/1, Gain1/1  "g"
  Constant1/1 -> Add/2
  Add/1 -> Gain2/1
  Gain2/1 -> Add1/2
  Gain3/1 -> Add1/3
  Constant/1 -> MinMax/1
  Fs/1 -> MinMax/2, sign/1
  MinMax/1 -> Divide2/1
  sign/1 -> Divide2/2
  Gain1/1 -> Add1/1
  Divide1/1 -> Add4/2
  Constant2/1 -> Add2/2
  v_rel/1 -> Abs1/1, Abs/1, sign1/1, Gain3/1  "v_rel"
  Abs1/1 -> Gain4/1
  Gain4/1 -> Math Function2/1
  Math Function2/1 -> Divide3/2, Add2/1
  sign1/1 -> Divide4/2
  Add4/1 -> Fd/1
  Add1/1 -> Divide4/1
  Divide4/1 -> Divide1/2
  Divide3/1 -> Add4/1
  Add2/1 -> Divide1/1
  Divide2/1 -> Divide3/1

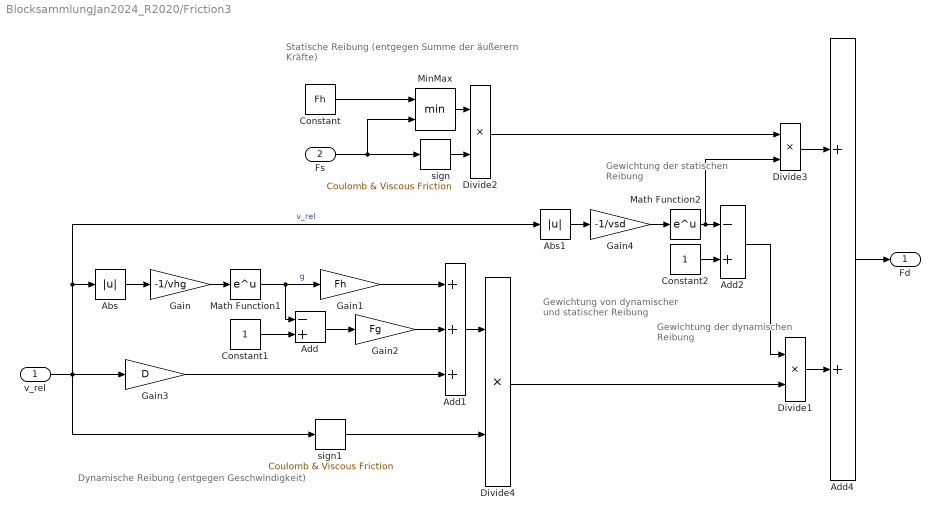
== system BlocksammlungJan2024_R2020/Friction3 ==
  note: Gewichtung von dynamischer
      |  und statischer Reibung
  note: Statische Reibung
      | (entgegen Summe der äußerern Kräfte)
  note: Dynamische Reibung (entgegen Geschwindigkeit)
  note: Gewichtung der
      | dynamischen Reibung
  note: Gewichtung der
      | statischen Reibung
  v_rel : Inport
  Fs : Inport  Port=2
  Abs : Abs
  Abs1 : Abs
  Add : Sum  Inputs=-+
  Add1 : Sum  Inputs=+++
  Add2 : Sum  Inputs=-+
  Add4 : Sum
  Constant : Constant  Value=Fh
  Constant1 : Constant
  Constant2 : Constant
  Divide{1..4} (4 alike) : Product  Inputs=**
  Gain : Gain  Gain=-1/vhg
  Gain1 : Gain  Gain=Fh
  Gain2 : Gain  Gain=Fg
  Gain3 : Gain  Gain=D
  Gain4 : Gain  Gain=-1/vsd
  Math Function1 : Math  SignedPower=on  SaturateOnIntegerOverflow=on
  Math Function2 : Math  SignedPower=on  SaturateOnIntegerOverflow=on
  MinMax : MinMax  Inputs=2
  sign : simulink/Discontinuities/Coulomb & Viscous Friction  offset=[1]  gain=0
  sign1 : simulink/Discontinuities/Coulomb & Viscous Friction  offset=[1]  gain=0
  Fd : Outport  VectorParamsAs1DForOutWhenUnconnected=off
  wires:
  Abs/1 -> Gain/1
  Gain/1 -> Math Function1/1
  Math Function1/1 -> Add/1, Gain1/1  "g"
  Constant1/1 -> Add/2
  Add/1 -> Gain2/1
  Gain2/1 -> Add1/2
  Gain3/1 -> Add1/3
  Constant/1 -> MinMax/1
  Fs/1 -> MinMax/2, sign/1
  MinMax/1 -> Divide2/1
  sign/1 -> Divide2/2
  Gain1/1 -> Add1/1
  Divide1/1 -> Add4/2
  Constant2/1 -> Add2/2
  v_rel/1 -> Abs1/1, Abs/1, sign1/1, Gain3/1  "v_rel"
  Abs1/1 -> Gain4/1
  Gain4/1 -> Math Function2/1
  Math Function2/1 -> Divide3/2, Add2/1
  sign1/1 -> Divide4/2
  Add4/1 -> Fd/1
  Add1/1 -> Divide4/1
  Divide4/1 -> Divide1/2
  Divide3/1 -> Add4/1
  Add2/1 -> Divide1/1
  Divide2/1 -> Divide3/1

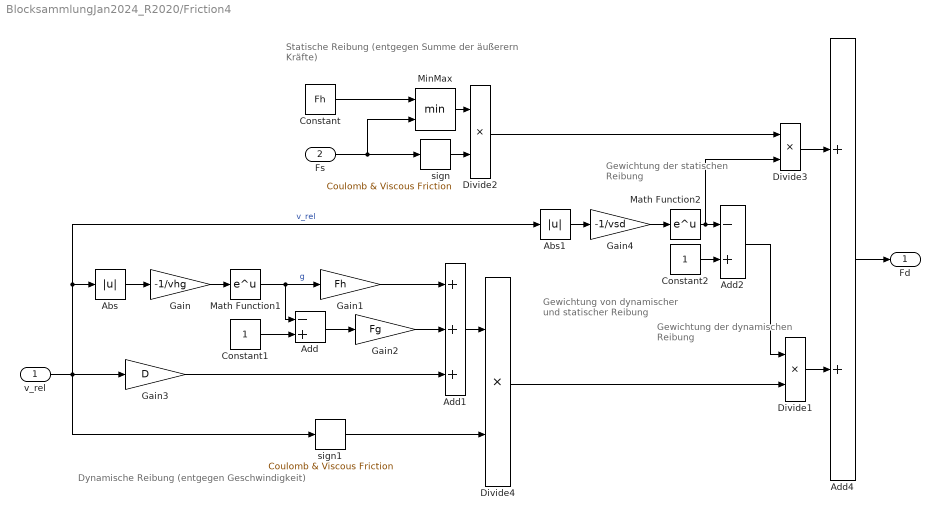
== system BlocksammlungJan2024_R2020/Friction4 ==
  note: Gewichtung von dynamischer
      |  und statischer Reibung
  note: Statische Reibung
      | (entgegen Summe der äußerern Kräfte)
  note: Dynamische Reibung (entgegen Geschwindigkeit)
  note: Gewichtung der
      | dynamischen Reibung
  note: Gewichtung der
      | statischen Reibung
  v_rel : Inport
  Fs : Inport  Port=2
  Abs : Abs
  Abs1 : Abs
  Add : Sum  Inputs=-+
  Add1 : Sum  Inputs=+++
  Add2 : Sum  Inputs=-+
  Add4 : Sum
  Constant : Constant  Value=Fh
  Constant1 : Constant
  Constant2 : Constant
  Divide{1..4} (4 alike) : Product  Inputs=**
  Gain : Gain  Gain=-1/vhg
  Gain1 : Gain  Gain=Fh
  Gain2 : Gain  Gain=Fg
  Gain3 : Gain  Gain=D
  Gain4 : Gain  Gain=-1/vsd
  Math Function1 : Math  SignedPower=on  SaturateOnIntegerOverflow=on
  Math Function2 : Math  SignedPower=on  SaturateOnIntegerOverflow=on
  MinMax : MinMax  Inputs=2
  sign : simulink/Discontinuities/Coulomb & Viscous Friction  offset=[1]  gain=0
  sign1 : simulink/Discontinuities/Coulomb & Viscous Friction  offset=[1]  gain=0
  Fd : Outport  VectorParamsAs1DForOutWhenUnconnected=off
  wires:
  Abs/1 -> Gain/1
  Gain/1 -> Math Function1/1
  Math Function1/1 -> Add/1, Gain1/1  "g"
  Constant1/1 -> Add/2
  Add/1 -> Gain2/1
  Gain2/1 -> Add1/2
  Gain3/1 -> Add1/3
  Constant/1 -> MinMax/1
  Fs/1 -> MinMax/2, sign/1
  MinMax/1 -> Divide2/1
  sign/1 -> Divide2/2
  Gain1/1 -> Add1/1
  Divide1/1 -> Add4/2
  Constant2/1 -> Add2/2
  v_rel/1 -> Abs1/1, Abs/1, sign1/1, Gain3/1  "v_rel"
  Abs1/1 -> Gain4/1
  Gain4/1 -> Math Function2/1
  Math Function2/1 -> Divide3/2, Add2/1
  sign1/1 -> Divide4/2
  Add4/1 -> Fd/1
  Add1/1 -> Divide4/1
  Divide4/1 -> Divide1/2
  Divide3/1 -> Add4/1
  Add2/1 -> Divide1/1
  Divide2/1 -> Divide3/1

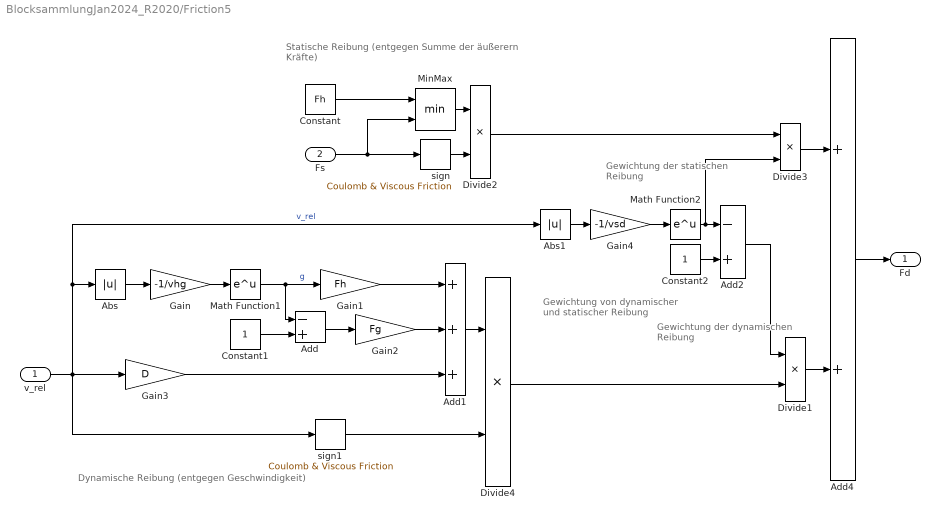
== system BlocksammlungJan2024_R2020/Friction5 ==
  note: Gewichtung von dynamischer
      |  und statischer Reibung
  note: Statische Reibung
      | (entgegen Summe der äußerern Kräfte)
  note: Dynamische Reibung (entgegen Geschwindigkeit)
  note: Gewichtung der
      | dynamischen Reibung
  note: Gewichtung der
      | statischen Reibung
  v_rel : Inport
  Fs : Inport  Port=2
  Abs : Abs
  Abs1 : Abs
  Add : Sum  Inputs=-+
  Add1 : Sum  Inputs=+++
  Add2 : Sum  Inputs=-+
  Add4 : Sum
  Constant : Constant  Value=Fh
  Constant1 : Constant
  Constant2 : Constant
  Divide{1..4} (4 alike) : Product  Inputs=**
  Gain : Gain  Gain=-1/vhg
  Gain1 : Gain  Gain=Fh
  Gain2 : Gain  Gain=Fg
  Gain3 : Gain  Gain=D
  Gain4 : Gain  Gain=-1/vsd
  Math Function1 : Math  SignedPower=on  SaturateOnIntegerOverflow=on
  Math Function2 : Math  SignedPower=on  SaturateOnIntegerOverflow=on
  MinMax : MinMax  Inputs=2
  sign : simulink/Discontinuities/Coulomb & Viscous Friction  offset=[1]  gain=0
  sign1 : simulink/Discontinuities/Coulomb & Viscous Friction  offset=[1]  gain=0
  Fd : Outport  VectorParamsAs1DForOutWhenUnconnected=off
  wires:
  Abs/1 -> Gain/1
  Gain/1 -> Math Function1/1
  Math Function1/1 -> Add/1, Gain1/1  "g"
  Constant1/1 -> Add/2
  Add/1 -> Gain2/1
  Gain2/1 -> Add1/2
  Gain3/1 -> Add1/3
  Constant/1 -> MinMax/1
  Fs/1 -> MinMax/2, sign/1
  MinMax/1 -> Divide2/1
  sign/1 -> Divide2/2
  Gain1/1 -> Add1/1
  Divide1/1 -> Add4/2
  Constant2/1 -> Add2/2
  v_rel/1 -> Abs1/1, Abs/1, sign1/1, Gain3/1  "v_rel"
  Abs1/1 -> Gain4/1
  Gain4/1 -> Math Function2/1
  Math Function2/1 -> Divide3/2, Add2/1
  sign1/1 -> Divide4/2
  Add4/1 -> Fd/1
  Add1/1 -> Divide4/1
  Divide4/1 -> Divide1/2
  Divide3/1 -> Add4/1
  Add2/1 -> Divide1/1
  Divide2/1 -> Divide3/1

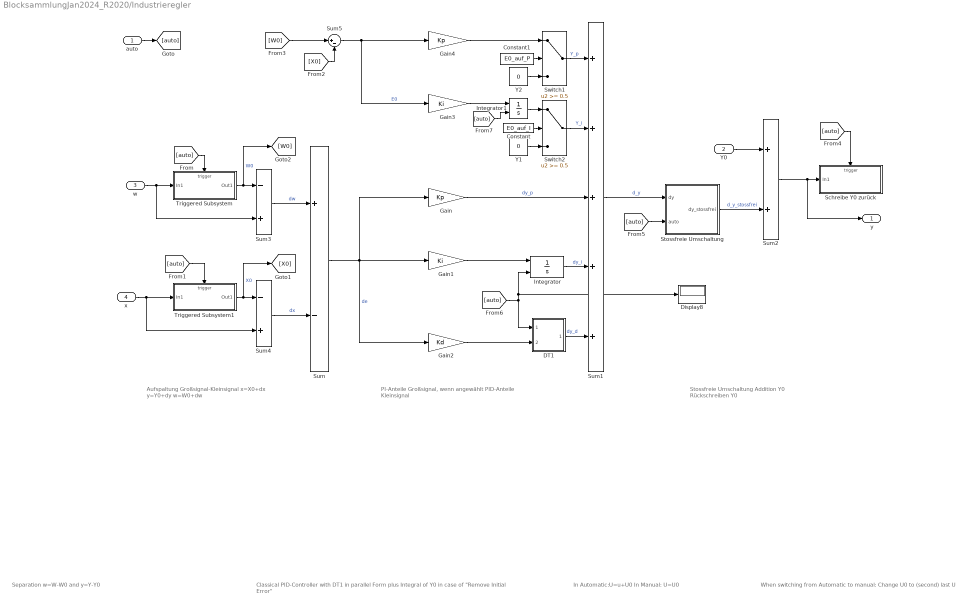
== system BlocksammlungJan2024_R2020/Industrieregler ==
  note: Stossfreie Umschaltung
      | Addition Y0
      | Rückschreiben Y0
  note: PI-Anteile Großsignal, wenn angewählt
      | PID-Anteile Kleinsignal
  note: Separation w=W-W0
      | and y=Y-Y0
  note: Classical PID-Controller with DT1 in parallel Form
      | plus Integral of Y0 in case of "Remove Initial Error"
  note: In Automatic:U=u+U0
      | In Manual: U=U0
  note: When switching from Automatic to manual:
      | Change U0 to (second) last U
  note: Aufspaltung Großsignal-Kleinsignal
      | x=X0+dx
      | y=Y0+dy
      | w=W0+dw
  auto : Inport
  Y0 : Inport  Port=2
  w : Inport  Port=3
  x : Inport  Port=4
  Constant : Constant  Value=E0_auf_I
  Constant1 : Constant  Value=E0_auf_P
  DT1 : Subsystem
  Display8 : Display
  Gain : Gain  Gain=Kp
  Gain1 : Gain  Gain=Ki
  Gain2 : Gain  Gain=Kd
  Gain3 : Gain  Gain=Ki
  Gain4 : Gain  Gain=Kp
  Integrator : Integrator  ExternalReset=rising
  Integrator1 : Integrator  ExternalReset=rising
  Schreibe Y0 zurück : Subsystem  TreatAsAtomicUnit=on
  Stossfreie Umschaltung : Subsystem
  Sum : Sum  Inputs=+-
  Sum1 : Sum  Inputs=+++++
  Sum2 : Sum
  Sum3 : Sum  Inputs=-+
  Sum4 : Sum  Inputs=-+
  Sum5 : Sum  Inputs=|+-
  Switch1 : Switch  Threshold=0.5
  Switch2 : Switch  Threshold=0.5
  Triggered Subsystem : Subsystem  TreatAsAtomicUnit=on
  Triggered Subsystem1 : Subsystem  TreatAsAtomicUnit=on
  Y1 : Constant  Value=0
  Y2 : Constant  Value=0
  y : Outport  VectorParamsAs1DForOutWhenUnconnected=off
  wires:
  [auto] -> Stossfreie Umschaltung/2(auto)
  Switch2/1 -> Sum1/2  "Y_i"
  [auto] -> Integrator1/2
  Y1/1 -> Switch2/3
  Constant/1 -> Switch2/2
  Integrator1/1 -> Switch2/1
  Gain3/1 -> Integrator1/1
  Sum5/1 -> Gain4/1, Gain3/1  "E0"
  Switch1/1 -> Sum1/1  "Y_p"
  Gain/1 -> Sum1/3  "dy_p"
  Integrator/1 -> Sum1/4  "dy_i"
  DT1/1(Out1) -> Sum1/5  "dy_d"
  Gain4/1 -> Switch1/1
  Y2/1 -> Switch1/3
  Constant1/1 -> Switch1/2
  [W0] -> Sum5/1
  Stossfreie Umschaltung/1(dy_stossfrei) -> Sum2/2  "d_y_stossfrei"
  Sum1/1 -> Stossfreie Umschaltung/1(dy)  "d_y"
  Gain2/1 -> DT1/2(kd_mal_de)
  [X0] -> Sum5/2
  Y0/1 -> Sum2/1
  auto/1 -> [auto]
  Sum/1 -> Gain1/1, Gain/1, Gain2/1  "de"
  Gain1/1 -> Integrator/1
  [auto] -> Triggered Subsystem1/Trigger
  [auto] -> Triggered Subsystem/Trigger
  Triggered Subsystem1/1(Out1) -> [X0], Sum4/1  "X0"
  Sum4/1 -> Sum/2  "dx"
  x/1 -> Triggered Subsystem1/1(In1), Sum4/2
  Triggered Subsystem/1(Out1) -> [W0], Sum3/1  "W0"
  Sum3/1 -> Sum/1  "dw"
  w/1 -> Triggered Subsystem/1(In1), Sum3/2
  [auto] -> Schreibe Y0 zurück/Trigger
  Sum2/1 -> y/1, Schreibe Y0 zurück/1(In1)
  [auto] -> DT1/1(auto), Integrator/2, Display8/1

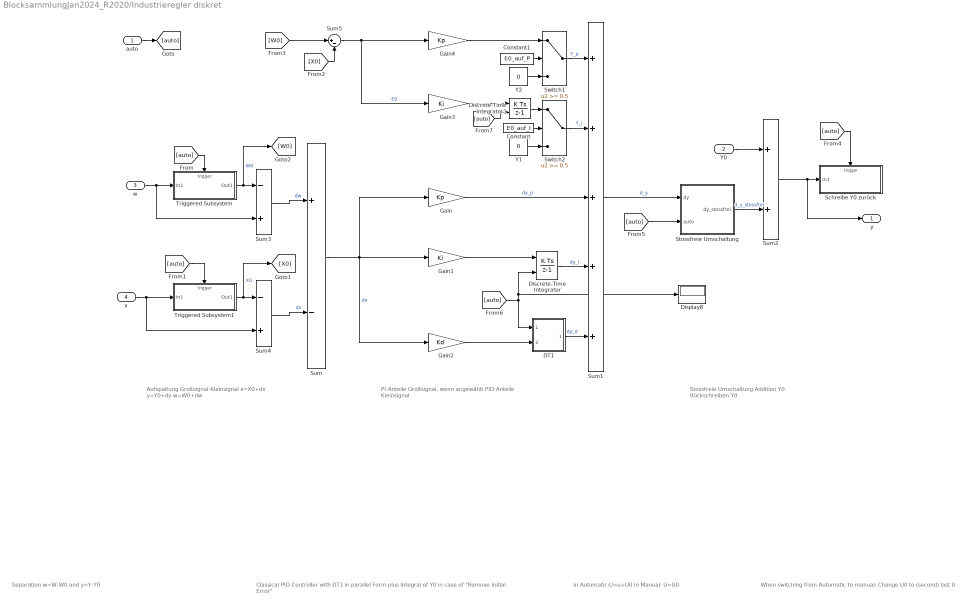
== system BlocksammlungJan2024_R2020/Industrieregler diskret ==
  note: Aufspaltung Großsignal-Kleinsignal
      | x=X0+dx
      | y=Y0+dy
      | w=W0+dw
  note: When switching from Automatic to manual:
      | Change U0 to (second) last U
  note: In Automatic:U=u+U0
      | In Manual: U=U0
  note: Classical PID-Controller with DT1 in parallel Form
      | plus Integral of Y0 in case of "Remove Initial Error"
  note: Separation w=W-W0
      | and y=Y-Y0
  note: PI-Anteile Großsignal, wenn angewählt
      | PID-Anteile Kleinsignal
  note: Stossfreie Umschaltung
      | Addition Y0
      | Rückschreiben Y0
  auto : Inport
  Y0 : Inport  Port=2
  w : Inport  Port=3
  x : Inport  Port=4
  Constant : Constant  Value=E0_auf_I
  Constant1 : Constant  Value=E0_auf_P
  DT1 : Subsystem
  Discrete-Time Integrator : DiscreteIntegrator  ExternalReset=rising  SampleTime=ta  ICPrevOutput=DiscIntNeverNeededParam  ICPrevScaledInput=DiscIntNeverNeededParam
  Discrete-Time Integrator1 : DiscreteIntegrator  ExternalReset=rising  SampleTime=ta  ICPrevOutput=DiscIntNeverNeededParam  ICPrevScaledInput=DiscIntNeverNeededParam
  Display8 : Display
  Gain : Gain  Gain=Kp
  Gain1 : Gain  Gain=Ki
  Gain2 : Gain  Gain=Kd
  Gain3 : Gain  Gain=Ki
  Gain4 : Gain  Gain=Kp
  Schreibe Y0 zurück : Subsystem  TreatAsAtomicUnit=on
  Stossfreie Umschaltung : Subsystem
  Sum : Sum  Inputs=+-
  Sum1 : Sum  Inputs=+++++
  Sum2 : Sum
  Sum3 : Sum  Inputs=-+
  Sum4 : Sum  Inputs=-+
  Sum5 : Sum  Inputs=|+-
  Switch1 : Switch  Threshold=0.5
  Switch2 : Switch  Threshold=0.5
  Triggered Subsystem : Subsystem  TreatAsAtomicUnit=on
  Triggered Subsystem1 : Subsystem  TreatAsAtomicUnit=on
  Y1 : Constant  Value=0
  Y2 : Constant  Value=0
  y : Outport  VectorParamsAs1DForOutWhenUnconnected=off
  wires:
  [auto] -> Discrete-Time Integrator/2, Display8/1, DT1/1(auto)
  Sum2/1 -> Schreibe Y0 zurück/1(In1), y/1
  [auto] -> Schreibe Y0 zurück/Trigger
  w/1 -> Sum3/2, Triggered Subsystem/1(In1)
  Sum3/1 -> Sum/1  "dw"
  Triggered Subsystem/1(Out1) -> Sum3/1, [W0]  "W0"
  x/1 -> Sum4/2, Triggered Subsystem1/1(In1)
  Sum4/1 -> Sum/2  "dx"
  Triggered Subsystem1/1(Out1) -> Sum4/1, [X0]  "X0"
  [auto] -> Triggered Subsystem/Trigger
  [auto] -> Triggered Subsystem1/Trigger
  Gain1/1 -> Discrete-Time Integrator/1
  Sum/1 -> Gain2/1, Gain/1, Gain1/1  "de"
  auto/1 -> [auto]
  Y0/1 -> Sum2/1
  [X0] -> Sum5/2
  Gain2/1 -> DT1/2(kd_mal_de)
  [W0] -> Sum5/1
  Constant1/1 -> Switch1/2
  Y2/1 -> Switch1/3
  Gain4/1 -> Switch1/1
  DT1/1(Out1) -> Sum1/5  "dy_d"
  Discrete-Time Integrator/1 -> Sum1/4  "dy_i"
  Gain/1 -> Sum1/3  "dy_p"
  Switch1/1 -> Sum1/1  "Y_p"
  Sum5/1 -> Gain3/1, Gain4/1  "E0"
  Gain3/1 -> Discrete-Time Integrator1/1
  Discrete-Time Integrator1/1 -> Switch2/1
  Constant/1 -> Switch2/2
  Y1/1 -> Switch2/3
  [auto] -> Discrete-Time Integrator1/2
  Switch2/1 -> Sum1/2  "Y_i"
  [auto] -> Stossfreie Umschaltung/2(auto)
  Stossfreie Umschaltung/1(dy_stossfrei) -> Sum2/2  "d_y_stossfrei"
  Sum1/1 -> Stossfreie Umschaltung/1(dy)  "d_y"

== system BlocksammlungJan2024_R2020/Kondensator ==
  i : Inport
  1dC : Gain  Gain=1/C
  Integrator : Integrator
  u : Outport  VectorParamsAs1DForOutWhenUnconnected=off
  wires:
  i/1 -> Integrator/1  "i"
  1dC/1 -> u/1  "u"
  Integrator/1 -> 1dC/1  "ii"

== system BlocksammlungJan2024_R2020/Kondensator1 ==
  u : Inport
  1dC : Gain  Gain=1/C
  Integrator : Integrator
  i : Outport  VectorParamsAs1DForOutWhenUnconnected=off
  wires:
  u/1 -> Integrator/1  "u"
  1dC/1 -> i/1  "i"
  Integrator/1 -> 1dC/1  "ui"

== system BlocksammlungJan2024_R2020/KondensatorMitDiff ==
  u : Inport
  C : Gain  Gain=C
  Derivative : Derivative
  i : Outport  VectorParamsAs1DForOutWhenUnconnected=off
  wires:
  u/1 -> Derivative/1  "u"
  C/1 -> i/1  "i"
  Derivative/1 -> C/1  "u'"

== system BlocksammlungJan2024_R2020/KondensatorMitDiff1 ==
  u : Inport
  C : Gain  Gain=C
  Derivative : Derivative
  i : Outport  VectorParamsAs1DForOutWhenUnconnected=off
  wires:
  u/1 -> Derivative/1  "u"
  C/1 -> i/1  "i"
  Derivative/1 -> C/1  "u'"

== system BlocksammlungJan2024_R2020/Laborstrecke ==
  Z : Inport
  Y : Inport  Port=2
  Strecke1_y : TransferFcn  Denominator=[2.6213e+003,492.8360,49.9349,1.2341]
  Strecke1_z : TransferFcn  Denominator=[-1.4728e3,-534.157,-137.5577,-4.4778]
  Sum : Sum  Inputs=|+-
  Sum1 : Sum  Inputs=|+-
  Sum2 : Sum  Inputs=--+
  X0 : Constant  Value=5.9
  Y0 : Constant  Value=5
  Z0 : Constant  Value=8.5
  X : Outport  VectorParamsAs1DForOutWhenUnconnected=off
  wires:
  Sum/1 -> Strecke1_y/1
  Y0/1 -> Sum/2
  Sum1/1 -> Strecke1_z/1
  Z0/1 -> Sum1/2
  Strecke1_z/1 -> Sum2/1
  Strecke1_y/1 -> Sum2/2
  X0/1 -> Sum2/3
  Z/1 -> Sum1/1
  Y/1 -> Sum/1
  Sum2/1 -> X/1  "X"

== system BlocksammlungJan2024_R2020/Masse ==
  F : Inport
  1/m : Gain  Gain=1/m
  Integrator : Integrator  InitialCondition=v0
  Integrator1 : Integrator  InitialCondition=s0
  s : Outport  VectorParamsAs1DForOutWhenUnconnected=off
  v : Outport  Port=2  VectorParamsAs1DForOutWhenUnconnected=off
  wires:
  1/m/1 -> Integrator/1
  Integrator/1 -> Integrator1/1, v/1
  F/1 -> 1/m/1
  Integrator1/1 -> s/1  "s"

== system BlocksammlungJan2024_R2020/Masse0 ==
  F : Inport
  1/m : Gain  Gain=1/m
  Integrator : Integrator  InitialCondition=v0
  Integrator1 : Integrator  InitialCondition=s0
  s : Outport  VectorParamsAs1DForOutWhenUnconnected=off
  wires:
  1/m/1 -> Integrator/1
  Integrator/1 -> Integrator1/1
  F/1 -> 1/m/1
  Integrator1/1 -> s/1  "s"

== system BlocksammlungJan2024_R2020/Masse1 ==
  F : Inport
  1/m : Gain  Gain=1/m
  Integrator : Integrator  InitialCondition=v0
  Integrator1 : Integrator  InitialCondition=s0
  s : Outport  VectorParamsAs1DForOutWhenUnconnected=off
  v : Outport  Port=2  VectorParamsAs1DForOutWhenUnconnected=off
  wires:
  1/m/1 -> Integrator/1
  Integrator/1 -> Integrator1/1, v/1
  F/1 -> 1/m/1
  Integrator1/1 -> s/1  "s"

== system BlocksammlungJan2024_R2020/Masse2 ==
  F : Inport
  1/m : Gain  Gain=1/m
  Integrator : Integrator  InitialCondition=v0
  Integrator1 : Integrator  InitialCondition=s0
  s : Outport  VectorParamsAs1DForOutWhenUnconnected=off
  v : Outport  Port=2  VectorParamsAs1DForOutWhenUnconnected=off
  wires:
  1/m/1 -> Integrator/1
  Integrator/1 -> Integrator1/1, v/1
  F/1 -> 1/m/1
  Integrator1/1 -> s/1  "s"

== system BlocksammlungJan2024_R2020/OP1 ==
  Plus : Inport
  Minus : Inport  Port=2
  Gain : Gain  Gain=k0
  Sum4 : Sum  Inputs=|+-
  Transfer Fcn : TransferFcn  Denominator=[1/2/pi/fg 1]
  u_a : Outport  VectorParamsAs1DForOutWhenUnconnected=off
  wires:
  Plus/1 -> Sum4/1
  Gain/1 -> u_a/1
  Sum4/1 -> Transfer Fcn/1
  Transfer Fcn/1 -> Gain/1
  Minus/1 -> Sum4/2

== system BlocksammlungJan2024_R2020/PID-Regler2 ==
  w : Inport
  x : Inport  Port=2
  Derivative6 : Derivative
  Integrator5 : Integrator
  Sum : Sum  Inputs=|+-
  Sum9 : Sum  Inputs=+++
  Transfer Fcn : TransferFcn  Denominator=[T 1]
  k_pr1 : Gain  Gain=Ki
  k_pr2 : Gain  Gain=Kp
  k_pr3 : Gain  Gain=Kd
  y : Outport  VectorParamsAs1DForOutWhenUnconnected=off
  wires:
  k_pr3/1 -> Sum9/3  "yd"
  k_pr1/1 -> Sum9/2  "yi"
  Transfer Fcn/1 -> Derivative6/1
  Integrator5/1 -> k_pr1/1
  Sum/1 -> k_pr2/1, Transfer Fcn/1, Integrator5/1
  k_pr2/1 -> Sum9/1  "yp"
  Derivative6/1 -> k_pr3/1
  w/1 -> Sum/1
  Sum9/1 -> y/1
  x/1 -> Sum/2
